simulink model "Bouncing2Simple"  (R2016a)
settings: Solver=VariableStepAuto  StartTime=0.0  StopTime=10.0  RelTol=1e-3
values from neighbouring files (symbols this model uses):
  k = 10    [BouncingScript.m]
libraries: dspsrcs4 x1
settings Model: Creator=Radu  LastModifiedBy=Radu

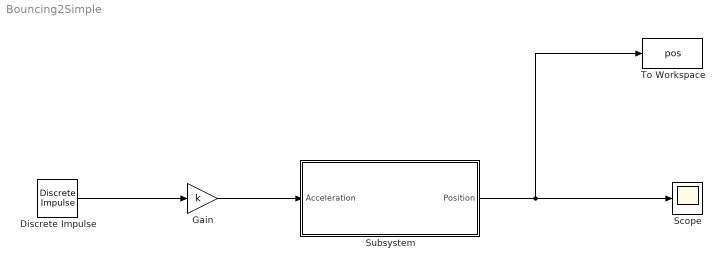
== system Bouncing2Simple ==
  Discrete Impulse : dspsrcs4/Discrete  Impulse  Delay=0  SampleTime=1  FrameSample=1  OutputFrames=off  dataType=double  isSigned=on  wordLen=16  udDataType=sfix(16)  fracBitsMode=Best precision  numFracBits=15  OutDataTypeStr=double  LastOutDataTypeStr=double
  Gain : Gain  Gain=k
  Scope : Scope
  Subsystem : Subsystem
  To Workspace : ToWorkspace  VariableName=pos  SaveFormat=Timeseries  SampleTime=-1
  wires:
  Subsystem/1("Position ") -> To Workspace/1, Scope/1
  Gain/1 -> Subsystem/1("Acceleration ")
  Discrete Impulse/1 -> Gain/1

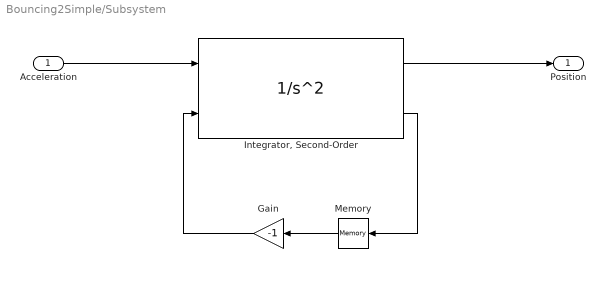
== system Bouncing2Simple/Subsystem ==
  "Acceleration " : Inport
  Gain : Gain  Gain=-1
  "Integrator, Second-Order" : SecondOrderIntegrator  ICX=0  LimitX=on  UpperLimitX=10  LowerLimitX=0  ICSourceDXDT=external  ReinitDXDTwhenXreachesSaturation=on
  Memory : Memory
  "Position " : Outport
  wires:
  Gain/1 -> "Integrator, Second-Order"/2
  "Integrator, Second-Order"/1 -> "Position "/1
  "Acceleration "/1 -> "Integrator, Second-Order"/1
  "Integrator, Second-Order"/2 -> Memory/1
  Memory/1 -> Gain/1
